simulink model "chorus"  (R2019a)
settings: Solver=VariableStepAuto  StartTime=0.0  StopTime=20  RelTol=1e-3
libraries: dspvision x1, dspobslib x1, dspsigops x1
settings Model: Creator=Ahmed  LastModifiedBy=Ahmed

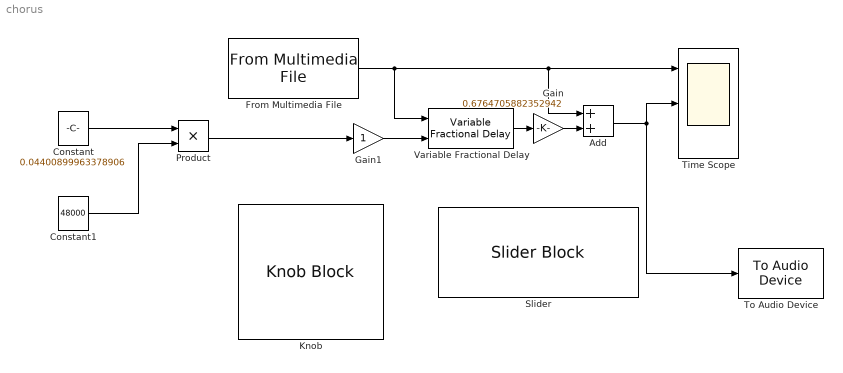
== system chorus ==
  Add : Sum
  Constant : Constant  Value=0.04400899963378906  VectorParams1D=off
  Constant1 : Constant  Value=48000  VectorParams1D=off
  From Multimedia File : dspvision/From Multimedia File  inputFilename=C:\Users\Ahmed\Nextcloud\L3\LU3EE105\Audio\Documents de TP et projet-20191118\Projet\tchai.wav  readRange=[1 Inf]  loop=on  numPlays=inf  outputStreams=Audio only  videoDataType=single  audioDataType=double  inheritSampleTime=on  userDefinedSampleTime=1/30  noAudioOutput=off  isIntensityVideo=off  fourcc=RGB  colorVideoFormat=Separate color signals  outputEOF=off  dataOrg=Column-major  audioFrameSize=1024  computeAudioFrameSize=off  outSamplingMode=Sample based
      settings: SourceProductName=DSP System Toolbox  SourceProductBaseCode=DS
  Gain : Gain  Gain=0.6764705882352942
  Gain1 : Gain
  Knob : KnobBlock  ScaleMin=0.02  ScaleMax=0.050000000000000003
  Product : Product
  Slider : SliderBlock  ScaleMax=1
  Time Scope : Scope  NumInputPorts=3
  To Audio Device : dspobslib/To Audio Device  deviceName=Default  inheritSampleRate=on  sampleRate=44100  deviceDatatype=Determine from input data type  autoBufferSize=on  bufferSize=4096  queueDuration=1.0  defaultOutputChannelMapping=on  outputChannelMapping=1:2  outputNumUnderrunSamples=off
      settings: SourceProductName=DSP System Toolbox  SourceProductBaseCode=DS
  Variable Fractional Delay : dspsigops/Variable Fractional Delay  mode=OBSOLETE  modeActive=Linear  L=4  FarrowL=4  R=10  alpha=1  dmax=100  InputProcessing=Columns as channels (frame based)  ic=0  noDFT=off  fallbackFIR=Clip to the minimum value necessary for centered kernel  fallbackFarrow=Clip to the minimum value necessary for centered kernel  roundingMode=Zero  overflowMode=off
      settings: SourceProductName=DSP System Toolbox  SourceProductBaseCode=DS
  wires:
  Add/1 -> To Audio Device/1, Time Scope/2
  Gain1/1 -> Variable Fractional Delay/2
  Constant/1 -> Product/1
  Variable Fractional Delay/1 -> Gain/1
  From Multimedia File/1 -> Variable Fractional Delay/1, Time Scope/1, Add/1
  Gain/1 -> Add/2
  Constant1/1 -> Product/2
  Product/1 -> Gain1/1
